simulink model "generador_signal"  (R2020a)
settings: Solver=VariableStepAuto  StartTime=0.0  StopTime=2  RelTol=1e-3
settings Model: Creator=HP  LastModifiedBy=HP

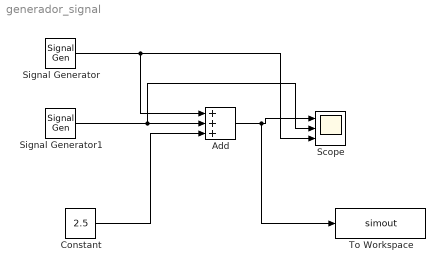
== system generador_signal ==
  Add : Sum  Inputs=+++
  Constant : Constant  Value=2.5
  Scope : Scope  NumInputPorts=3
  Signal Generator : SignalGenerator  Amplitude=2  Frequency=0.5
  Signal Generator1 : SignalGenerator  Amplitude=0.3  Frequency=40
  To Workspace : ToWorkspace  VariableName=simout  SampleTime=0.01
  wires:
  Signal Generator/1 -> Scope/3, Add/1
  Signal Generator1/1 -> Scope/2, Add/2
  Constant/1 -> Add/3
  Add/1 -> To Workspace/1, Scope/1
